simulink model "windEmulatorStep4_WECSim"  (R2025b)
settings: Solver=ode14x  StartTime=0  StopTime=400  FixedStep=Ts  MaxStep=0.01  RelTol=1e-3
values from neighbouring files (symbols this model uses):
  A = 1.0    (= 1)    [initStep4.m]
  absEncoderCountsToRad = 1/2^20*2*pi    (= 5.99211245268e-06)    [initStep4.m]
  acs800CtrlStruct =     [windEmulatorBusDefs.mat]
  acs800DcBusVoltsScaling = 1    [initStep4.m]
  acs800FreqScaling = 1/100    (= 0.01)    [initStep4.m]
  acs800PowerScaling = Gen_PowerScaling    (= 14.9109)    [initStep4.m]
  acs800SignalStruct =     [windEmulatorBusDefs.mat]
  acs800SpeedNomEng = 1500    [initStep4.m]
  acs800SpeedNomFb = 20000    [initStep4.m]
  acs800SpeedScaling = 1500/20000    (= 0.075)    [initStep4.m]
  acs800TempScaling = 1/10    (= 0.1)    [initStep4.m]
  acs800TorqueNomEng = 100    [initStep4.m]
  acs800TorqueNomFb = 10000    [initStep4.m]
  acs800TorqueScaling = acs800TorqueRating/10000    (= 0.008035933)    [initStep4.m]
  acs880CtrlStruct =     [windEmulatorBusDefs.mat]
  acs880FreqScaling = 60/20000    (= 0.003)    [initStep4.m]
  acs880MotorCurrentScaling = 100/10000    (= 0.01)    [initStep4.m]
  acs880MotorVoltsScaling = 1    [initStep4.m]
  acs880PowerScaling = 100*hp2W/10000    (= 7.457)    [initStep4.m]
  acs880RatedTorque = 80.494    [initStep4.m]
  acs880RateLimFalling = -10000    [initStep4.m]
  acs880RateLimRising = 10000    [initStep4.m]
  acs880SetpointLimLower = -0.975*acs880RatedTorque    (= -78.48165)    [initStep4.m]
  acs880SetpointLimUpper = 0.975*acs880RatedTorque    (= 78.48165)    [initStep4.m]
  acs880SignalStruct =     [windEmulatorBusDefs.mat]
  acs880SpeedPILimLo = -0.975*acs880RatedTorque    (= -78.48165)    [initStep4.m]
  acs880SpeedPILimUp = 0.975*acs880RatedTorque    (= 78.48165)    [initStep4.m]
  acs880SpeedScaling = 2000/20000    (= 0.1)    [initStep4.m]
  acs880TorqueFieldbusScale = 10000    [initStep4.m]
  acs880TorqueScaling = acs880RatedTorque/acs880TorqueFieldbusScale    (= 0.0080494)    [initStep4.m]
  acs880TorqueSetpointScaling = 100    [initStep4.m]
  bar2pa = 1e5    (= 100000)    [initStep4.m]
  belowMinPGain = 1/200    (= 0.005)    [initStep4.m]
  ctrlModeTorque = logical(true)    [init.m]    (also in initStep1.m; initStep2.m; initStep3.m; initStep4.m)
  ctrlSignal1 = squeeze(hptoSignalsData.Values.ctrlSignal1.Data)    [postProcessingStep2.m]
  ctrlSignal2 = squeeze(hptoSignalsData.Values.ctrlSignal2.Data)    [postProcessingStep2.m]
  deadBandController = boolean(false)    [initStep4.m]
  deadbandTorqueSlewRate = 300    [initStep4.m]
  Dm_max = 40    [initStep4.m]
  EffMechMax = 0.93    [initStep4.m]
  EffMechMin = 0.79    [initStep4.m]
  excForce_N = squeeze(hptoCtrlData.Values.excForce_N.Data)    [postProcessingStep2.m]
  expCtrlStruct =     [windEmulatorBusDefs.mat]
  FactorEff = psi2pa*cc2m3*(1/rev2rad)    (= 0.00109733470463)    [initStep4.m]
  fromFileSpeedSlewRate = 250    [initStep4.m]
  fromFileTorqueSlewRate = 25    [initStep4.m]
  futekTorqueScale = -1/(2^31)*10/5*100    (= -9.31322574615e-08)    [initStep4.m]
  genMaxTorque = 0.8*ratedTorque    (= 64.3952)    [initStep3.m]    (also in initStep4.m = 78.48165)
  genTorqueCmd_Nm = squeeze(hptoSignalsData.Values.genTorqueCmd_Nm.Data)    [postProcessingStep2.m]
  hbmCtScale = 1/1.5    (= 0.666666666667)    [initStep4.m]
  hbmPowerStruct =     [windEmulatorBusDefs.mat]
  hptoCtrlStruct =     [windEmulatorBusDefs.mat]
  hptoSignalStruct =     [windEmulatorBusDefs.mat]
  invPowerStruct =     [windEmulatorBusDefs.mat]
  lpm2m3ps = 1/m3ps2lpm    (= 1.66666666667e-05)    [initStep4.m]
  minPressureRef_psi = 1000    [initStep4.m]
  minTorqueRef_Nm = (minPressureRef_psi*psi2pa)*(Dm_max*cc2m3*(1/rev2rad))    (= 43.8933881851)    [initStep4.m]
  motorSpeed_rpm = squeeze(acs880SignalsData.Values.motorSpeed_rpm.Data)    [postProcessingStep2.m]
  nPreDrop = 2900    [initStep4.m]
  nPreDropMin = 725    [initStep4.m]
  psi2bar = 1/bar2psi    (= 0.0689475729318)    [initStep4.m]
  radps2rpm = 60/(2*pi)    (= 9.54929658551)    [initStep2.m]    (also in initStep4.m)
  rpm2radps = 2*pi/60    (= 0.10471975512)    [initStep4.m]
  runCounter = squeeze(hptoCtrlData.Values.runCounter.Data)    [postProcessingStep2.m]
  shaftSignalStruct =     [windEmulatorBusDefs.mat]
  sidCtrlStruct =     [windEmulatorBusDefs.mat]
  sidDataCaseCounter = sidData.experimentData.count    [initStep4.m]
  sidDataSpeed_rpm = sidData.experimentData.wShaft_rpm    [initStep4.m]
  sidDataTorque_Nm = sidData.experimentData.torqueShaft_Nm    [initStep4.m]
  sidInfoStruct =     [windEmulatorBusDefs.mat]
  T = 4    [initStep4.m]
  targetOmega = 2000/60*2*pi    (= 209.439510239)    [initStep2.m]    (also in initStep3.m; initStep4.m)
  time = hptoCtrlData.Values.runCounter.Time    [postProcessingStep2.m]
  TorqueLoadMax = 75    [initStep4.m]
  Ts = 1/250    (= 0.004)    [initStep4.m]
undefined symbols (not defined in the file or in its folder): absEncoderCounts, absEncoderPosition_rad, absEncoderSpeed_rpm, absEncoderStatus1, absEncoderStatus2, absEncoderTurns, accVolHP, acs800Torque_Nm, acs800TorqueSetpoint_Nm, acs880SpeedSetpoint_rpm, acs880Torque_Nm, body, constraint, crankLength, ctrlWord, dcBusVoltage_V, DiscIntNeverNeededParam, Dmax, excShaftSpeed_rpm, excShaftTorque_Nm, expType, expTypeEnum, frequency_Hz, fromFileCaseCounter, genPumpFlow_lpm, genShaftSpeed_rpm, genShaftSpeedRef, genSpeedActual, hmOutputShafTorque_Nm, iGainGen, m3persecond2lpm, motorCurrent_A, motorTorque_Nm, motorVoltage_V, offsetLength, pa2psi, pGainGen, pressure_bar, PressureControl, pto, radsec2rpm, ramp, resetHilIntegrator, resetSidIntegrator, rodLength, runHil, runSid, shaftPower_W, sidType, sidTypeEnum, SpeedControl, speedCtrlReset, speedRef_rpm, state, statusWord, stepCounter, temperature, torqueActual_Nm, TorqueInputControl, torqueSetpoint_Nm ... (+1)
libraries: slrealtimeethercatlib x118, fl_lib x81, nesl_utility x45, sh_lib x18, slrealtimeloglib x13, dspstat3 x5, slpidlib x4, simulink_extras x4, cstblocks x3, dspindex x3, WECSim_Lib_Body_Elements x2, simulink x2
(part 2 of 6)

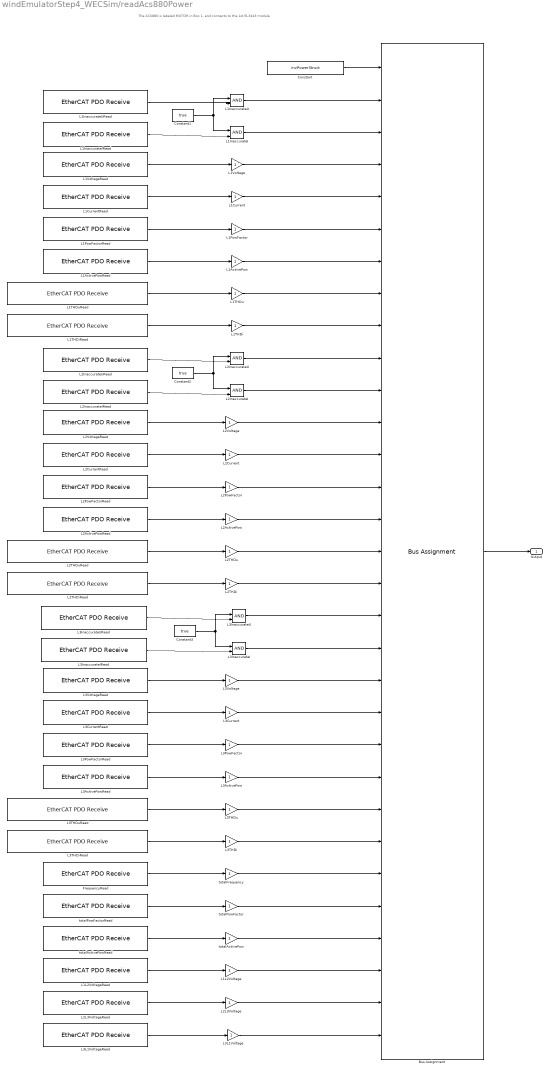
== system windEmulatorStep4_WECSim/readAcs880Power ==
  note: The ACS880 is labeled MOTOR in Box 1, and connects to the 1st EL3443 module
  Bus Assignment : BusAssignment  AssignedSignals=L1InaccurateU,L1InaccurateI,L1Voltage,L1Current,L1PowFactor,L1ActivePow,L1THDu,L1THDi,L2InaccurateU,L2InaccurateI,L2Voltage,L2Current,L2PowFactor,L2ActivePow,L2THDu,L2THDi,L3InaccurateU,L3InaccurateI,L3Voltage,L3Current,L3PowFactor,L3ActivePow,L3THDu,L3THDi,Frequency,TotalPowFactor,TotalActivePow,L1L2Voltage,L2L3Voltage,L3L1Volage
  Constant : Constant  Value=invPowerStruct  OutDataTypeStr=Bus: invPowerBus
  Constant1 : Constant  Value=true  OutDataTypeStr=boolean
  Constant2 : Constant  Value=true  OutDataTypeStr=boolean
  Constant3 : Constant  Value=true  OutDataTypeStr=boolean
  FrequencyRead : slrealtimeethercatlib/EtherCAT PDO Receive  Priority=2  sig_name=POW_EL3443_01.Total Basic.Frequency  sig_offset=2280  sig_type=single  type_size=32  sig_dim=1  device_id=0  sample_time=0.004000
  L1ActivePow : Gain  OutDataTypeStr=double
  L1ActivePowRead : slrealtimeethercatlib/EtherCAT PDO Receive  Priority=2  sig_name=POW_EL3443_01.L1 Power.Active Power  sig_offset=1064  sig_type=single  type_size=32  sig_dim=1  device_id=0  sample_time=0.004000
  L1Current : Gain  OutDataTypeStr=double
  L1CurrentRead : slrealtimeethercatlib/EtherCAT PDO Receive  Priority=2  sig_name=POW_EL3443_01.L1 Basic.Current  sig_offset=1032  sig_type=single  type_size=32  sig_dim=1  device_id=0  sample_time=0.004000
  L1InaccurateI : Logic  IconShape=distinctive  AllPortsSameDT=off  OutDataTypeStr=boolean
  L1InaccurateIRead : slrealtimeethercatlib/EtherCAT PDO Receive  Priority=2  sig_name=POW_EL3443_01.L1 Status.Inaccurate Current  sig_offset=988  sig_type=boolean  type_size=1  sig_dim=1  device_id=0  sample_time=0.004000
  L1InaccurateU : Logic  IconShape=distinctive  AllPortsSameDT=off  OutDataTypeStr=boolean
  L1InaccurateURead : slrealtimeethercatlib/EtherCAT PDO Receive  Priority=2  sig_name=POW_EL3443_01.L1 Status.Inaccurate Voltage  sig_offset=987  sig_type=boolean  type_size=1  sig_dim=1  device_id=0  sample_time=0.004000
  L1L2Voltage : Gain  OutDataTypeStr=double
  L1L2VoltageRead : slrealtimeethercatlib/EtherCAT PDO Receive  Priority=2  sig_name=POW_EL3443_01.Total L-L Voltage.L1-L2 Voltage  sig_offset=2600  sig_type=single  type_size=32  sig_dim=1  device_id=0  sample_time=0.004000
  L1PowFactor : Gain  OutDataTypeStr=double
  L1PowFactorRead : slrealtimeethercatlib/EtherCAT PDO Receive  Priority=2  sig_name=POW_EL3443_01.L1 Power.Power Factor  sig_offset=1160  sig_type=single  type_size=32  sig_dim=1  device_id=0  sample_time=0.004000
  L1THDi : Gain  OutDataTypeStr=double
  L1THDiRead : slrealtimeethercatlib/EtherCAT PDO Receive  Priority=2  sig_name=POW_EL3443_01.L1 Advanced.Current Total Harmonic Distortion  sig_offset=1336  sig_type=single  type_size=32  sig_dim=1  device_id=0  sample_time=0.004000
  L1THDu : Gain  OutDataTypeStr=double
  L1THDuRead : slrealtimeethercatlib/EtherCAT PDO Receive  Priority=2  sig_name=POW_EL3443_01.L1 Advanced.Voltage Total Harmonic Distortion  sig_offset=1272  sig_type=single  type_size=32  sig_dim=1  device_id=0  sample_time=0.004000
  L1Voltage : Gain  OutDataTypeStr=double
  L1VoltageRead : slrealtimeethercatlib/EtherCAT PDO Receive  Priority=2  sig_name=POW_EL3443_01.L1 Basic.Voltage  sig_offset=1000  sig_type=single  type_size=32  sig_dim=1  device_id=0  sample_time=0.004000
  L2ActivePow : Gain  OutDataTypeStr=double
  L2ActivePowRead : slrealtimeethercatlib/EtherCAT PDO Receive  Priority=2  sig_name=POW_EL3443_01.L2 Power.Active Power  sig_offset=1480  sig_type=single  type_size=32  sig_dim=1  device_id=0  sample_time=0.004000
  L2Current : Gain  OutDataTypeStr=double
  L2CurrentRead : slrealtimeethercatlib/EtherCAT PDO Receive  Priority=2  sig_name=POW_EL3443_01.L2 Basic.Current  sig_offset=1448  sig_type=single  type_size=32  sig_dim=1  device_id=0  sample_time=0.004000
  L2InaccurateI : Logic  IconShape=distinctive  AllPortsSameDT=off  OutDataTypeStr=boolean
  L2InaccurateIRead : slrealtimeethercatlib/EtherCAT PDO Receive  Priority=2  sig_name=POW_EL3443_01.L2 Status.Inaccurate Current  sig_offset=1404  sig_type=boolean  type_size=1  sig_dim=1  device_id=0  sample_time=0.004000
  L2InaccurateU : Logic  IconShape=distinctive  AllPortsSameDT=off  OutDataTypeStr=boolean
  L2InaccurateURead : slrealtimeethercatlib/EtherCAT PDO Receive  Priority=2  sig_name=POW_EL3443_01.L2 Status.Inaccurate Voltage  sig_offset=1403  sig_type=boolean  type_size=1  sig_dim=1  device_id=0  sample_time=0.004000
  L2L3Voltage : Gain  OutDataTypeStr=double
  L2L3VoltageRead : slrealtimeethercatlib/EtherCAT PDO Receive  Priority=2  sig_name=POW_EL3443_01.Total L-L Voltage.L2-L3 Voltage  sig_offset=2632  sig_type=single  type_size=32  sig_dim=1  device_id=0  sample_time=0.004000
  L2PowFactor : Gain  OutDataTypeStr=double
  L2PowFactorRead : slrealtimeethercatlib/EtherCAT PDO Receive  Priority=2  sig_name=POW_EL3443_01.L2 Power.Power Factor  sig_offset=1576  sig_type=single  type_size=32  sig_dim=1  device_id=0  sample_time=0.004000
  L2THDi : Gain  OutDataTypeStr=double
  L2THDiRead : slrealtimeethercatlib/EtherCAT PDO Receive  Priority=2  sig_name=POW_EL3443_01.L2 Advanced.Current Total Harmonic Distortion  sig_offset=1752  sig_type=single  type_size=32  sig_dim=1  device_id=0  sample_time=0.004000
  L2THDu : Gain  OutDataTypeStr=double
  L2THDuRead : slrealtimeethercatlib/EtherCAT PDO Receive  Priority=2  sig_name=POW_EL3443_01.L2 Advanced.Voltage Total Harmonic Distortion  sig_offset=1688  sig_type=single  type_size=32  sig_dim=1  device_id=0  sample_time=0.004000
  L2Voltage : Gain  OutDataTypeStr=double
  L2VoltageRead : slrealtimeethercatlib/EtherCAT PDO Receive  Priority=2  sig_name=POW_EL3443_01.L2 Basic.Voltage  sig_offset=1416  sig_type=single  type_size=32  sig_dim=1  device_id=0  sample_time=0.004000
  L3ActivePow : Gain  OutDataTypeStr=double
  L3ActivePowRead : slrealtimeethercatlib/EtherCAT PDO Receive  Priority=2  sig_name=POW_EL3443_01.L3 Power.Active Power  sig_offset=1896  sig_type=single  type_size=32  sig_dim=1  device_id=0  sample_time=0.004000
  L3Current : Gain  OutDataTypeStr=double
  L3CurrentRead : slrealtimeethercatlib/EtherCAT PDO Receive  Priority=2  sig_name=POW_EL3443_01.L3 Basic.Current  sig_offset=1864  sig_type=single  type_size=32  sig_dim=1  device_id=0  sample_time=0.004000
  L3InaccurateI : Logic  IconShape=distinctive  AllPortsSameDT=off  OutDataTypeStr=boolean
  L3InaccurateIRead : slrealtimeethercatlib/EtherCAT PDO Receive  Priority=2  sig_name=POW_EL3443_01.L3 Status.Inaccurate Current  sig_offset=1820  sig_type=boolean  type_size=1  sig_dim=1  device_id=0  sample_time=0.004000
  L3InaccurateU : Logic  IconShape=distinctive  AllPortsSameDT=off  OutDataTypeStr=boolean
  L3InaccurateURead : slrealtimeethercatlib/EtherCAT PDO Receive  Priority=2  sig_name=POW_EL3443_01.L3 Status.Inaccurate Voltage  sig_offset=1819  sig_type=boolean  type_size=1  sig_dim=1  device_id=0  sample_time=0.004000
  L3L1Voltage : Gain  OutDataTypeStr=double
  L3L1VoltageRead : slrealtimeethercatlib/EtherCAT PDO Receive  Priority=2  sig_name=POW_EL3443_01.Total L-L Voltage.L3-L1 Voltage  sig_offset=2664  sig_type=single  type_size=32  sig_dim=1  device_id=0  sample_time=0.004000
  L3PowFactor : Gain  OutDataTypeStr=double
  L3PowFactorRead : slrealtimeethercatlib/EtherCAT PDO Receive  Priority=2  sig_name=POW_EL3443_01.L3 Power.Power Factor  sig_offset=1992  sig_type=single  type_size=32  sig_dim=1  device_id=0  sample_time=0.004000
  L3THDi : Gain  OutDataTypeStr=double
  L3THDiRead : slrealtimeethercatlib/EtherCAT PDO Receive  Priority=2  sig_name=POW_EL3443_01.L3 Advanced.Current Total Harmonic Distortion  sig_offset=2168  sig_type=single  type_size=32  sig_dim=1  device_id=0  sample_time=0.004000
  L3THDu : Gain  OutDataTypeStr=double
  L3THDuRead : slrealtimeethercatlib/EtherCAT PDO Receive  Priority=2  sig_name=POW_EL3443_01.L3 Advanced.Voltage Total Harmonic Distortion  sig_offset=2104  sig_type=single  type_size=32  sig_dim=1  device_id=0  sample_time=0.004000
  L3Voltage : Gain  OutDataTypeStr=double
  L3VoltageRead : slrealtimeethercatlib/EtherCAT PDO Receive  Priority=2  sig_name=POW_EL3443_01.L3 Basic.Voltage  sig_offset=1832  sig_type=single  type_size=32  sig_dim=1  device_id=0  sample_time=0.004000
  totalActivePow : Gain  OutDataTypeStr=double
  totalActivePowRead : slrealtimeethercatlib/EtherCAT PDO Receive  Priority=2  sig_name=POW_EL3443_01.Total Active.Active Power  sig_offset=2376  sig_type=single  type_size=32  sig_dim=1  device_id=0  sample_time=0.004000
  totalFrequency : Gain  OutDataTypeStr=double
  totalPowFactor : Gain  OutDataTypeStr=double
  totalPowFactorRead : slrealtimeethercatlib/EtherCAT PDO Receive  Priority=2  sig_name=POW_EL3443_01.Total Basic.Power Factor  sig_offset=2312  sig_type=single  type_size=32  sig_dim=1  device_id=0  sample_time=0.004000
  Output : Outport  OutDataTypeStr=Bus: invPowerBus
  wires:
  L1VoltageRead/1 -> L1Voltage/1
  Constant/1 -> Bus Assignment/1
  Bus Assignment/1 -> Output/1
  L1Voltage/1 -> Bus Assignment/4
  L1CurrentRead/1 -> L1Current/1
  L1Current/1 -> Bus Assignment/5
  L1PowFactorRead/1 -> L1PowFactor/1
  L1PowFactor/1 -> Bus Assignment/6
  L1ActivePowRead/1 -> L1ActivePow/1
  L1ActivePow/1 -> Bus Assignment/7
  L1THDuRead/1 -> L1THDu/1
  L1THDu/1 -> Bus Assignment/8
  L1THDi/1 -> Bus Assignment/9
  L1THDiRead/1 -> L1THDi/1
  L2THDiRead/1 -> L2THDi/1
  L2THDi/1 -> Bus Assignment/17
  L2THDu/1 -> Bus Assignment/16
  L2THDuRead/1 -> L2THDu/1
  L2ActivePow/1 -> Bus Assignment/15
  L2ActivePowRead/1 -> L2ActivePow/1
  L2PowFactor/1 -> Bus Assignment/14
  L2PowFactorRead/1 -> L2PowFactor/1
  L2Current/1 -> Bus Assignment/13
  L2CurrentRead/1 -> L2Current/1
  L2Voltage/1 -> Bus Assignment/12
  L2VoltageRead/1 -> L2Voltage/1
  L3VoltageRead/1 -> L3Voltage/1
  L3Voltage/1 -> Bus Assignment/20
  L3CurrentRead/1 -> L3Current/1
  L3Current/1 -> Bus Assignment/21
  L3PowFactorRead/1 -> L3PowFactor/1
  L3PowFactor/1 -> Bus Assignment/22
  L3ActivePowRead/1 -> L3ActivePow/1
  L3ActivePow/1 -> Bus Assignment/23
  L3THDuRead/1 -> L3THDu/1
  L3THDu/1 -> Bus Assignment/24
  L3THDi/1 -> Bus Assignment/25
  L3THDiRead/1 -> L3THDi/1
  Constant1/1 -> L1InaccurateU/1, L1InaccurateI/1
  L1InaccurateU/1 -> Bus Assignment/2
  L1InaccurateURead/1 -> L1InaccurateU/2
  L1InaccurateI/1 -> Bus Assignment/3
  L1InaccurateIRead/1 -> L1InaccurateI/2
  Constant2/1 -> L2InaccurateU/1, L2InaccurateI/1
  L2InaccurateURead/1 -> L2InaccurateU/2
  L2InaccurateI/1 -> Bus Assignment/11
  L2InaccurateIRead/1 -> L2InaccurateI/2
  L2InaccurateU/1 -> Bus Assignment/10
  L3InaccurateU/1 -> Bus Assignment/18
  L3InaccurateI/1 -> Bus Assignment/19
  L3InaccurateIRead/1 -> L3InaccurateI/2
  Constant3/1 -> L3InaccurateU/1, L3InaccurateI/1
  L3InaccurateURead/1 -> L3InaccurateU/2
  FrequencyRead/1 -> totalFrequency/1
  totalFrequency/1 -> Bus Assignment/26
  totalPowFactorRead/1 -> totalPowFactor/1
  totalPowFactor/1 -> Bus Assignment/27
  totalActivePowRead/1 -> totalActivePow/1
  totalActivePow/1 -> Bus Assignment/28
  L1L2VoltageRead/1 -> L1L2Voltage/1
  L1L2Voltage/1 -> Bus Assignment/29
  L2L3Voltage/1 -> Bus Assignment/30
  L2L3VoltageRead/1 -> L2L3Voltage/1
  L3L1VoltageRead/1 -> L3L1Voltage/1
  L3L1Voltage/1 -> Bus Assignment/31

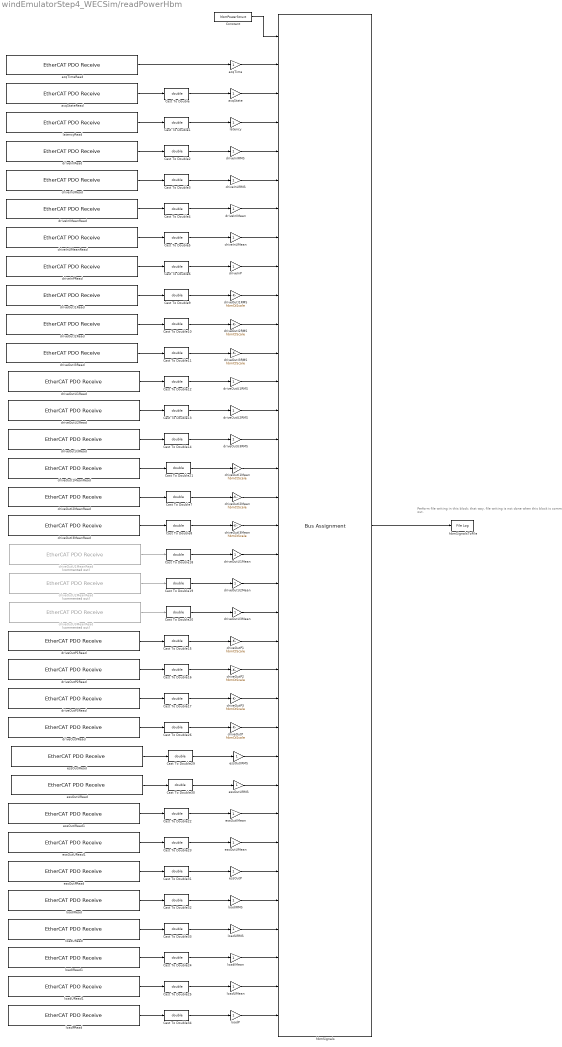
== system windEmulatorStep4_WECSim/readPowerHbm ==
  note: Perform file writing in this block; that way, file writing is not done when this block is commented out.
  Cast To Double{,1..26,29..34} (33 alike) : DataTypeConversion  OutDataTypeStr=double  SaturateOnIntegerOverflow=off  RndMeth=Floor
  Constant : Constant  Value=hbmPowerStruct  OutDataTypeStr=Bus: hbmPowerBus
  acqState : Gain  OutDataTypeStr=double
  acqStateRead : slrealtimeethercatlib/EtherCAT PDO Receive  Priority=2  sig_name=HBM_Power_Analyzer_01.AcquisitionState.AcquisitionState_S  sig_offset=4504  sig_type=uint8  type_size=8  sig_dim=1  device_id=0  sample_time=0.004000
  acqTime : Gain  OutDataTypeStr=double
  acqTimeRead : slrealtimeethercatlib/EtherCAT PDO Receive  Priority=2  sig_name=HBM_Power_Analyzer_01.AcquisitionTime.AcquisitionTime_V  sig_offset=4512  sig_type=double  type_size=64  sig_dim=1  device_id=0  sample_time=0.004000
  driveInIMean : Gain  OutDataTypeStr=double
  driveInIMeanRead : slrealtimeethercatlib/EtherCAT PDO Receive  Priority=2  sig_name=HBM_Power_Analyzer_01.Drive.in.i_mean.Drive.in.i_mean_V  sig_offset=4784  sig_type=single  type_size=32  sig_dim=1  device_id=0  sample_time=0.004000
  driveInIRMS : Gain  OutDataTypeStr=double
  driveInIRead : slrealtimeethercatlib/EtherCAT PDO Receive  Priority=2  sig_name=HBM_Power_Analyzer_01.Drive.in.I.Drive.in.I_V  sig_offset=4704  sig_type=single  type_size=32  sig_dim=1  device_id=0  sample_time=0.004000
  driveInP : Gain  OutDataTypeStr=double
  driveInPRead : slrealtimeethercatlib/EtherCAT PDO Receive  Priority=2  sig_name=HBM_Power_Analyzer_01.Drive.in.P.Drive.in.P_V  sig_offset=5104  sig_type=single  type_size=32  sig_dim=1  device_id=0  sample_time=0.004000
  driveInUMean : Gain  OutDataTypeStr=double
  driveInUMeanRead : slrealtimeethercatlib/EtherCAT PDO Receive  Priority=2  sig_name=HBM_Power_Analyzer_01.Drive.in.u_mean.Drive.in.u_mean_V  sig_offset=4824  sig_type=single  type_size=32  sig_dim=1  device_id=0  sample_time=0.004000
  driveInURMS : Gain  OutDataTypeStr=double
  driveInURead : slrealtimeethercatlib/EtherCAT PDO Receive  Priority=2  sig_name=HBM_Power_Analyzer_01.Drive.in.U.Drive.in.U_V  sig_offset=4744  sig_type=single  type_size=32  sig_dim=1  device_id=0  sample_time=0.004000
  driveOutI1Mean : Gain  Gain=hbmCtScale  OutDataTypeStr=double
  driveOutI1MeanRead : slrealtimeethercatlib/EtherCAT PDO Receive  Priority=2  sig_name=HBM_Power_Analyzer_01.Drive.out.i1_mean.Drive.out.i1_mean_V  sig_offset=5664  sig_type=single  type_size=32  sig_dim=1  device_id=0  sample_time=0.004000
  driveOutI1RMS : Gain  Gain=hbmCtScale  OutDataTypeStr=double
  driveOutI1Read : slrealtimeethercatlib/EtherCAT PDO Receive  Priority=2  sig_name=HBM_Power_Analyzer_01.Drive.out.I_1.Drive.out.I_1_V  sig_offset=4864  sig_type=single  type_size=32  sig_dim=1  device_id=0  sample_time=0.004000
  driveOutI2Mean : Gain  Gain=hbmCtScale  OutDataTypeStr=double
  driveOutI2MeanRead : slrealtimeethercatlib/EtherCAT PDO Receive  Priority=2  sig_name=HBM_Power_Analyzer_01.Drive.out.i2_mean.Drive.out.i2_mean_V  sig_offset=5704  sig_type=single  type_size=32  sig_dim=1  device_id=0  sample_time=0.004000
  driveOutI2RMS : Gain  Gain=hbmCtScale  OutDataTypeStr=double
  driveOutI2Read : slrealtimeethercatlib/EtherCAT PDO Receive  Priority=2  sig_name=HBM_Power_Analyzer_01.Drive.out.I_2.Drive.out.I_2_V  sig_offset=4904  sig_type=single  type_size=32  sig_dim=1  device_id=0  sample_time=0.004000
  driveOutI3Mean : Gain  Gain=hbmCtScale  OutDataTypeStr=double
  driveOutI3MeanRead : slrealtimeethercatlib/EtherCAT PDO Receive  Priority=2  sig_name=HBM_Power_Analyzer_01.Drive.out.i3_mean.Drive.out.i3_mean_V  sig_offset=5744  sig_type=single  type_size=32  sig_dim=1  device_id=0  sample_time=0.004000
  driveOutI3RMS : Gain  Gain=hbmCtScale  OutDataTypeStr=double
  driveOutI3Read : slrealtimeethercatlib/EtherCAT PDO Receive  Priority=2  sig_name=HBM_Power_Analyzer_01.Drive.out.I_3.Drive.out.I_3_V  sig_offset=5144  sig_type=single  type_size=32  sig_dim=1  device_id=0  sample_time=0.004000
  driveOutP{,1..3} (4 alike) : Gain  Gain=hbmCtScale  OutDataTypeStr=double
  driveOutP1Read : slrealtimeethercatlib/EtherCAT PDO Receive  Priority=2  sig_name=HBM_Power_Analyzer_01.Drive.out.P_1.Drive.out.P_1_V  sig_offset=5304  sig_type=single  type_size=32  sig_dim=1  device_id=0  sample_time=0.004000
  driveOutP2Read : slrealtimeethercatlib/EtherCAT PDO Receive  Priority=2  sig_name=HBM_Power_Analyzer_01.Drive.out.P_2.Drive.out.P_2_V  sig_offset=5344  sig_type=single  type_size=32  sig_dim=1  device_id=0  sample_time=0.004000
  driveOutP3Read : slrealtimeethercatlib/EtherCAT PDO Receive  Priority=2  sig_name=HBM_Power_Analyzer_01.Drive.out.P_3.Drive.out.P_3_V  sig_offset=5384  sig_type=single  type_size=32  sig_dim=1  device_id=0  sample_time=0.004000
  driveOutPRead : slrealtimeethercatlib/EtherCAT PDO Receive  Priority=2  sig_name=HBM_Power_Analyzer_01.Drive.out.P.Drive.out.P_V  sig_offset=5904  sig_type=single  type_size=32  sig_dim=1  device_id=0  sample_time=0.004000
  driveOutU1Mean : Gain  OutDataTypeStr=double
  driveOutU1MeanRead : slrealtimeethercatlib/EtherCAT PDO Receive  Priority=2  Commented=on  sig_name=HBM_Power_Analyzer_01.Drive_out.u1_mean.Drive_out.u1_mean_V  sig_offset=8208  sig_type=single  type_size=32  sig_dim=1  device_id=0  sample_time=0.001000
  driveOutU1RMS : Gain  OutDataTypeStr=double
  driveOutU1Read : slrealtimeethercatlib/EtherCAT PDO Receive  Priority=2  sig_name=HBM_Power_Analyzer_01.Drive.out.U_1.Drive.out.U_1_V  sig_offset=5184  sig_type=single  type_size=32  sig_dim=1  device_id=0  sample_time=0.004000
  driveOutU2Mean : Gain  OutDataTypeStr=double
  driveOutU2MeanRead : slrealtimeethercatlib/EtherCAT PDO Receive  Priority=2  Commented=on  sig_name=HBM_Power_Analyzer_01.Drive_out.u2_mean.Drive_out.u2_mean_V  sig_offset=8408  sig_type=single  type_size=32  sig_dim=1  device_id=0  sample_time=0.001000
  driveOutU2RMS : Gain  OutDataTypeStr=double
  driveOutU2Read : slrealtimeethercatlib/EtherCAT PDO Receive  Priority=2  sig_name=HBM_Power_Analyzer_01.Drive.out.U_2.Drive.out.U_2_V  sig_offset=5224  sig_type=single  type_size=32  sig_dim=1  device_id=0  sample_time=0.004000
  driveOutU3Mean : Gain  OutDataTypeStr=double
  driveOutU3MeanRead : slrealtimeethercatlib/EtherCAT PDO Receive  Priority=2  Commented=on  sig_name=HBM_Power_Analyzer_01.Drive_out.u3_mean.Drive_out.u3_mean_V  sig_offset=8448  sig_type=single  type_size=32  sig_dim=1  device_id=0  sample_time=0.001000
  driveOutU3RMS : Gain  OutDataTypeStr=double
  driveOutU3Read : slrealtimeethercatlib/EtherCAT PDO Receive  Priority=2  sig_name=HBM_Power_Analyzer_01.Drive.out.U_3.Drive.out.U_3_V  sig_offset=5264  sig_type=single  type_size=32  sig_dim=1  device_id=0  sample_time=0.004000
  essOutIMean : Gain  OutDataTypeStr=double
  essOutIRMS : Gain  OutDataTypeStr=double
  essOutIRead : slrealtimeethercatlib/EtherCAT PDO Receive  Priority=2  sig_name=HBM_Power_Analyzer_01.ESS.out1.I.ESS.out1.I_V  sig_offset=4624  sig_type=single  type_size=32  sig_dim=1  device_id=0  sample_time=0.004000
  essOutIRead1 : slrealtimeethercatlib/EtherCAT PDO Receive  Priority=2  sig_name=HBM_Power_Analyzer_01.ESS.out1.i_mean.ESS.out1.i_mean_V  sig_offset=5064  sig_type=single  type_size=32  sig_dim=1  device_id=0  sample_time=0.004000
  essOutP : Gain  OutDataTypeStr=double
  essOutPRead : slrealtimeethercatlib/EtherCAT PDO Receive  Priority=2  sig_name=HBM_Power_Analyzer_01.ESS.out1.P.ESS.out1.P_V  sig_offset=4944  sig_type=single  type_size=32  sig_dim=1  device_id=0  sample_time=0.004000
  essOutUMean : Gain  OutDataTypeStr=double
  essOutURMS : Gain  OutDataTypeStr=double
  essOutURead : slrealtimeethercatlib/EtherCAT PDO Receive  Priority=2  sig_name=HBM_Power_Analyzer_01.ESS.out1.U.ESS.out1.U_V  sig_offset=4664  sig_type=single  type_size=32  sig_dim=1  device_id=0  sample_time=0.004000
  essOutURead1 : slrealtimeethercatlib/EtherCAT PDO Receive  Priority=2  sig_name=HBM_Power_Analyzer_01.ESS.out1.u_mean.ESS.out1.u_mean_V  sig_offset=5544  sig_type=single  type_size=32  sig_dim=1  device_id=0  sample_time=0.004000
  hbmSignals : BusAssignment  AssignedSignals=acqTime,acqState,latency,driveInIRMS,driveInURMS,driveInIMean,driveInUMean,driveInP,driveOutI1RMS,driveOutI2RMS,driveOutI3RMS,driveOutU1RMS,driveOutU2RMS,driveOutU3RMS,driveOutI1Mean,driveOutI2Mean,driveOutI3Mean,driveOutU1Mean,driveOutU2Mean,driveOutU3Mean,driveOutP1,driveOutP2,driveOutP3,driveOutP,essOutIRMS,essOutURMS,essOutIMean,essOutUMean,essOutP,loadIRMS,loadURMS,loadIMean,loadUMean,loadP
  hbmSignalsToFile : slrealtimeloglib/File Log  decimation=fileDecimation  inputProcessing=Elements as channels (sample based)
  latency : Gain  OutDataTypeStr=double
  latencyRead : slrealtimeethercatlib/EtherCAT PDO Receive  Priority=2  sig_name=HBM_Power_Analyzer_01.Latency.Latency_V  sig_offset=4584  sig_type=single  type_size=32  sig_dim=1  device_id=0  sample_time=0.004000
  loadIMean : Gain  OutDataTypeStr=double
  loadIRMS : Gain  OutDataTypeStr=double
  loadIRead : slrealtimeethercatlib/EtherCAT PDO Receive  Priority=2  sig_name=HBM_Power_Analyzer_01.Load.in1.I.Load.in1.I_V  sig_offset=5424  sig_type=single  type_size=32  sig_dim=1  device_id=0  sample_time=0.004000
  loadIRead1 : slrealtimeethercatlib/EtherCAT PDO Receive  Priority=2  sig_name=HBM_Power_Analyzer_01.Load.in1.i_mean.Load.in1.i_mean_V  sig_offset=5584  sig_type=single  type_size=32  sig_dim=1  device_id=0  sample_time=0.004000
  loadP : Gain  OutDataTypeStr=double
  loadPRead : slrealtimeethercatlib/EtherCAT PDO Receive  Priority=2  sig_name=HBM_Power_Analyzer_01.Load.in1.P.Load.in1.P_V  sig_offset=5504  sig_type=single  type_size=32  sig_dim=1  device_id=0  sample_time=0.004000
  loadUMean : Gain  OutDataTypeStr=double
  loadURMS : Gain  OutDataTypeStr=double
  loadURead : slrealtimeethercatlib/EtherCAT PDO Receive  Priority=2  sig_name=HBM_Power_Analyzer_01.Load.in1.U.Load.in1.U_V  sig_offset=5464  sig_type=single  type_size=32  sig_dim=1  device_id=0  sample_time=0.004000
  loadURead1 : slrealtimeethercatlib/EtherCAT PDO Receive  Priority=2  sig_name=HBM_Power_Analyzer_01.Load.in1.u_mean.Load.in1.u_mean_V  sig_offset=5624  sig_type=single  type_size=32  sig_dim=1  device_id=0  sample_time=0.004000
  wires:
  acqTimeRead/1 -> acqTime/1
  acqTime/1 -> hbmSignals/2
  Constant/1 -> hbmSignals/1
  hbmSignals/1 -> hbmSignalsToFile/1
  Cast To Double/1 -> acqState/1
  acqState/1 -> hbmSignals/3
  latency/1 -> hbmSignals/4
  Cast To Double1/1 -> latency/1
  driveInIRead/1 -> Cast To Double2/1
  Cast To Double2/1 -> driveInIRMS/1
  driveInURead/1 -> Cast To Double3/1
  Cast To Double3/1 -> driveInURMS/1
  driveInIMeanRead/1 -> Cast To Double4/1
  Cast To Double4/1 -> driveInIMean/1
  driveInUMeanRead/1 -> Cast To Double5/1
  Cast To Double5/1 -> driveInUMean/1
  driveInPRead/1 -> Cast To Double6/1
  Cast To Double6/1 -> driveInP/1
  driveOutI1Read/1 -> Cast To Double9/1
  Cast To Double9/1 -> driveOutI1RMS/1
  driveOutI1RMS/1 -> hbmSignals/10
  driveOutI2Read/1 -> Cast To Double10/1
  Cast To Double10/1 -> driveOutI2RMS/1
  driveOutI2RMS/1 -> hbmSignals/11
  driveOutI3Read/1 -> Cast To Double11/1
  Cast To Double11/1 -> driveOutI3RMS/1
  driveOutI3RMS/1 -> hbmSignals/12
  driveOutU1Read/1 -> Cast To Double12/1
  Cast To Double12/1 -> driveOutU1RMS/1
  driveOutU1RMS/1 -> hbmSignals/13
  driveOutU2Read/1 -> Cast To Double13/1
  Cast To Double13/1 -> driveOutU2RMS/1
  driveOutU2RMS/1 -> hbmSignals/14
  driveOutU3Read/1 -> Cast To Double14/1
  Cast To Double14/1 -> driveOutU3RMS/1
  driveOutU3RMS/1 -> hbmSignals/15
  driveOutP1Read/1 -> Cast To Double15/1
  Cast To Double15/1 -> driveOutP1/1
  driveOutP1/1 -> hbmSignals/22
  driveOutP2Read/1 -> Cast To Double16/1
  Cast To Double16/1 -> driveOutP2/1
  driveOutP2/1 -> hbmSignals/23
  driveOutP3Read/1 -> Cast To Double17/1
  Cast To Double17/1 -> driveOutP3/1
  driveOutP3/1 -> hbmSignals/24
  driveOutPRead/1 -> Cast To Double26/1
  Cast To Double26/1 -> driveOutP/1
  driveOutP/1 -> hbmSignals/25
  essOutIRead/1 -> Cast To Double29/1
  Cast To Double29/1 -> essOutIRMS/1
  essOutURead/1 -> Cast To Double30/1
  Cast To Double30/1 -> essOutURMS/1
  essOutPRead/1 -> Cast To Double31/1
  Cast To Double31/1 -> essOutP/1
  essOutP/1 -> hbmSignals/30
  loadIRead/1 -> Cast To Double32/1
  Cast To Double32/1 -> loadIRMS/1
  loadURead/1 -> Cast To Double33/1
  Cast To Double33/1 -> loadURMS/1
  loadURMS/1 -> hbmSignals/32
  loadPRead/1 -> Cast To Double34/1
  Cast To Double34/1 -> loadP/1
  loadP/1 -> hbmSignals/35
  acqStateRead/1 -> Cast To Double/1
  latencyRead/1 -> Cast To Double1/1
  driveInIRMS/1 -> hbmSignals/5
  driveInURMS/1 -> hbmSignals/6
  driveInIMean/1 -> hbmSignals/7
  driveInUMean/1 -> hbmSignals/8
  driveInP/1 -> hbmSignals/9
  Cast To Double18/1 -> driveOutU1Mean/1
  driveOutI2MeanRead/1 -> Cast To Double7/1
  Cast To Double7/1 -> driveOutI2Mean/1
  driveOutU2MeanRead/1 -> Cast To Double19/1
  Cast To Double20/1 -> driveOutU3Mean/1
  driveOutI3MeanRead/1 -> Cast To Double8/1
  driveOutU1MeanRead/1 -> Cast To Double18/1
  driveOutU3MeanRead/1 -> Cast To Double20/1
  Cast To Double8/1 -> driveOutI3Mean/1
  driveOutI1MeanRead/1 -> Cast To Double21/1
  Cast To Double19/1 -> driveOutU2Mean/1
  Cast To Double21/1 -> driveOutI1Mean/1
  driveOutU3Mean/1 -> hbmSignals/21
  driveOutU2Mean/1 -> hbmSignals/20
  driveOutU1Mean/1 -> hbmSignals/19
  driveOutI3Mean/1 -> hbmSignals/18
  driveOutI2Mean/1 -> hbmSignals/17
  driveOutI1Mean/1 -> hbmSignals/16
  loadIRMS/1 -> hbmSignals/31
  essOutIRMS/1 -> hbmSignals/26
  essOutURMS/1 -> hbmSignals/27
  essOutIMean/1 -> hbmSignals/28
  essOutUMean/1 -> hbmSignals/29
  Cast To Double23/1 -> essOutUMean/1
  Cast To Double22/1 -> essOutIMean/1
  essOutURead1/1 -> Cast To Double23/1
  essOutIRead1/1 -> Cast To Double22/1
  loadUMean/1 -> hbmSignals/34
  loadURead1/1 -> Cast To Double25/1
  Cast To Double24/1 -> loadIMean/1
  loadIMean/1 -> hbmSignals/33
  loadIRead1/1 -> Cast To Double24/1
  Cast To Double25/1 -> loadUMean/1

== system windEmulatorStep4_WECSim/readShaftSignals ==
  note: Note: why is conversion to uint8 needed?
  Bus Assignment : BusAssignment  AssignedSignals=torqueActual_Nm,absEncoderCounts,absEncoderTurns,absEncoderPosition_rad,absEncoderSpeed_rpm,absEncoderStatus1,absEncoderStatus2
  Cast To Double : DataTypeConversion  OutDataTypeStr=double  SaturateOnIntegerOverflow=off  RndMeth=Floor
  Cast To Double1 : DataTypeConversion  OutDataTypeStr=uint8  SaturateOnIntegerOverflow=off  RndMeth=Floor
  Cast To Double2 : DataTypeConversion  OutDataTypeStr=uint8  SaturateOnIntegerOverflow=off  RndMeth=Floor
  Constant : Constant  Value=shaftSignalStruct  OutDataTypeStr=Bus: shaftSignalBus
  Demux : Demux  Outputs=2
  EtherCAT PDO Receive7 : slrealtimeethercatlib/EtherCAT PDO Receive  Priority=2  sig_name=InstA_EL5001_01.SSI Inputs.Status  sig_offset=936  sig_type=uint8  type_size=8  sig_dim=2  device_id=0  sample_time=0.004000
  Gain : Gain  Gain=futekTorqueScale
  countsToRads : Subsystem
  posToVel : simulink/Discrete/Discrete Derivative  gainval=1.0  ICPrevScaledInput=0.0  OutMin=[]  OutMax=[]  OutDataType=fixdt(1, 16)  OutScaling=2^-10  DoSatur=off
  rad/s->rpm : Gain  Gain=radps2rpm
  readEncoderCounter : slrealtimeethercatlib/EtherCAT PDO Receive  Priority=2  sig_name=InstA_EL5001_01.SSI Inputs.Counter value  sig_offset=952  sig_type=uint32  type_size=32  sig_dim=1  device_id=0  sample_time=0.004000
  readTorqueInput : slrealtimeethercatlib/EtherCAT PDO Receive  Priority=2  sig_name=InstA_EL3602_01.AI Inputs Channel 1.Value  sig_offset=856  sig_type=int32  type_size=32  sig_dim=1  device_id=0  sample_time=0.004000
  shaftSignals : Outport  OutDataTypeStr=Bus: shaftSignalBus
  wires:
  Bus Assignment/1 -> shaftSignals/1
  Constant/1 -> Bus Assignment/1
  readTorqueInput/1 -> Cast To Double/1
  Gain/1 -> Bus Assignment/2
  Demux/1 -> Cast To Double1/1
  Cast To Double/1 -> Gain/1
  Cast To Double1/1 -> Bus Assignment/7
  Demux/2 -> Cast To Double2/1
  Cast To Double2/1 -> Bus Assignment/8
  EtherCAT PDO Receive7/1 -> Demux/1  "encoderStatus"
  readEncoderCounter/1 -> countsToRads/1(rawCounts), Bus Assignment/3
  countsToRads/2(pos_rad) -> posToVel/1, Bus Assignment/5
  rad/s->rpm/1 -> Bus Assignment/6
  posToVel/1 -> rad/s->rpm/1
  countsToRads/1(turns) -> Bus Assignment/4

== system windEmulatorStep4_WECSim/sidCtrl ==
  expCtrl : Inport  OutDataTypeStr=Bus: expCtrlBus
  acs880Signals : Inport  Port=2  OutDataTypeStr=Bus: acs880SignalBus
  acs800Signals : Inport  Port=3  OutDataTypeStr=Bus: acs800SignalBus
  inportSpeed_rpm : Inport  Port=4
  inportTorque_Nm : Inport  Port=5
  inportCaseCounter : Inport  Port=6
  Bus Assignment : BusAssignment  AssignedSignals=acs800Torque_Nm,acs880Torque_Nm
  Bus Selector : BusSelector  OutputSignals=motorSpeed_rpm
  Bus Selector1 : BusSelector  OutputSignals=resetSidIntegrator
  Constant : Constant  Value=sidCtrlStruct  OutDataTypeStr=Bus: sidCtrlBus
  Constant1 : Constant  Value=acs880SpeedPILimUp
  Constant2 : Constant  Value=acs880SpeedPILimLo
  PID Controller : slpidlib/PID Controller  Controller=PI  Form=Parallel  TimeDomain=Continuous-time  UseExternalTs=off  SampleTime=-1  IntegratorMethod=Forward Euler  FilterMethod=Forward Euler  ControllerParametersSource=external  P=1  I=1  UseKiTs=off  D=0  UseExternalDerivativeSource=off  N=100  UseFilter=on  TunerSelectOption=Transfer Function Based (PID Tuner App)  InitialConditionSource=internal  InitialConditionForIntegrator=0  InitialConditionForFilter=0  DifferentiatorICPrevScaledInput=0  ExternalReset=level  TrackingMode=off  Kt=1  LimitOutput=on  SatLimitsSource=external  UpperSaturationLimit=inf  LowerSaturationLimit=-inf  LinearizeAsGain=on  AntiWindupMode=none  Kb=1  LimitIntegrator=off  UpperIntegratorSaturationLimit=inf  LowerIntegratorSaturationLimit=-inf  POutMin=[]  POutMax=[]  IOutMin=[]  IOutMax=[]  DOutMin=[]  DOutMax=[]  NOutMin=[]  NOutMax=[]  SumOutMin=[]  SumOutMax=[]  SaturationOutMin=[]  SaturationOutMax=[]  PParamMin=[]  PParamMax=[]  IParamMin=[]  IParamMax=[]  DParamMin=[]  DParamMax=[]  NParamMin=[]  NParamMax=[]  KbParamMin=[]  KbParamMax=[]  KtParamMin=[]  KtParamMax=[]  KbOutMin=[]  KbOutMax=[]  KtOutMin=[]  KtOutMax=[]  IntegratorOutMin=[]  IntegratorOutMax=[]  FilterOutMin=[]  FilterOutMax=[]  SumI1OutMin=[]  SumI1OutMax=[]  SumI2OutMin=[]  SumI2OutMax=[]  SumI3OutMin=[]  SumI3OutMax=[]  SumI4OutMin=[]  SumI4OutMax=[]  SumDOutMin=[]  SumDOutMax=[]  DifferentiatorOutMin=[]  DifferentiatorOutMax=[]  FilterDiffOutCoefMin=[]  FilterDiffOutCoefMax=[]  ReciprocalOutMin=[]  ReciprocalOutMax=[]  SumDenOutMin=[]  SumDenOutMax=[]  SumNumOutMin=[]  SumNumOutMax=[]  DivideOutMin=[]  DivideOutMax=[]  UdiffTsProdOutMin=[]  UdiffTsProdOutMax=[]  NTsProdOutMin=[]  NTsProdOutMax=[]  UintegralTsProdOutMin=[]  UintegralTsProdOutMax=[]  UngainTsProdOutMin=[]  UngainTsProdOutMax=[]  ClampingZeroOutDataTypeStr=Inherit: Inherit via back propagation  ClampingZeroOutMin=[]  ClampingZeroOutMax=[]  FilterDenConstantOutDataTypeStr=Inherit: Inherit via back propagation  FilterDenConstantOutMin=[]  FilterDenConstantOutMax=[]  PCopyOutDataTypeStr=Inherit: Inherit via back propagation  PCopyOutMin=[]  PCopyOutMax=[]  NCopyOutDataTypeStr=Inherit: Inherit via back propagation  NCopyOutMin=[]  NCopyOutMax=[]  IntegratorContinuousStateAttributes=''  IntegratorStateMustResolveToSignalObject=off  IntegratorRTWStateStorageClass=Auto  FilterContinuousStateAttributes=''  FilterStateMustResolveToSignalObject=off  FilterRTWStateStorageClass=Auto  ParallelPVariant=ExternalParameters  IdealPVariant=Disabled  IVariant=ExternalParameters  DVariant=Disabled  IntegratorVariant=Continuous  SatVariant=External  AWVariant=Passthrough  PCopyVariant=Disabled  TRVariant=Disabled  FdbkBlocksVariant=Forward  IdealPFdbkVariant=Disabled  SatFdbkVariant=Disabled  DerivativeFilterVariant=Disabled  NVariant=Disabled  NCopyVariant=Disabled_SignalSpec  FilterICVariant=Disabled  IntegratorICVariant=InternalICs  ExternalResetVariant=ExternalReset  TRSumVariant=Passthrough  SumFdbkVariant=Disabled  SumVariant=Sum_PI  TsampFilterVariant=InternalTs  TsampNgainVariant=Passthrough  TsampIntegralVariant=Disabled_SignalSpec  ExternalSaturationOutDataTypeStr=Inherit: Same as second input  DerivativeSourceVariant=Disabled  PreIntVariant=InternalPreInt
  Sum : Sum  Inputs=|+-
  Terminator1 : Terminator
  acs880SpeedIGain : Constant  Value=0
  acs880SpeedPGain : Constant  Value=0
  setpointGenerator : Subsystem
  sidCtrlSignals : Outport  OutDataTypeStr=Bus: sidCtrlBus
  sidInfoSignals : Outport  Port=2  OutDataTypeStr=Bus: sidInfoBus
  wires:
  Constant/1 -> Bus Assignment/1
  Bus Assignment/1 -> sidCtrlSignals/1
  acs800Signals/1 -> Terminator1/1
  acs880Signals/1 -> Bus Selector/1
  setpointGenerator/2(acs880SpeedSetpoint_rpm) -> Sum/1
  Bus Selector/1 -> Sum/2  "<motorSpeed_rpm>"
  setpointGenerator/1(acs800TorqueSetpoint_Nm) -> Bus Assignment/2
  Sum/1 -> PID Controller/1
  PID Controller/1 -> Bus Assignment/3
  acs880SpeedPGain/1 -> PID Controller/2
  acs880SpeedIGain/1 -> PID Controller/3
  expCtrl/1 -> Bus Selector1/1, setpointGenerator/1(expCtrl)
  Bus Selector1/1 -> PID Controller/4  "<resetSidIntegrator>"
  Constant1/1 -> PID Controller/5
  Constant2/1 -> PID Controller/6
  setpointGenerator/3(sidInfoSignals) -> sidInfoSignals/1
  inportSpeed_rpm/1 -> setpointGenerator/2(inportSpeed_rpm)
  inportTorque_Nm/1 -> setpointGenerator/3(inportTorque_Nm)
  inportCaseCounter/1 -> setpointGenerator/4(inportCaseCounter)

== system windEmulatorStep4_WECSim/writeAcs800Pdos ==
  note: Set to zero; we are in torque control.
  acs800CtrlSignals : Inport  OutDataTypeStr=Bus: acs800CtrlBus
  ACS800ConvertREF1 : Subsystem  mask{EngineeringValue=acs800SpeedNomEng, FieldbusValue=acs800SpeedNomFb}
      mask prompts: EngineeringValue "Engineering units nominal value:"; FieldbusValue "Fieldbus nominal value:"
  ACS800ConvertREF2 : Subsystem  mask{EngineeringValue=acs800TorqueNomEng, FieldbusValue=acs800TorqueNomFb}
      mask prompts: EngineeringValue "Engineering units nominal value:"; FieldbusValue "Fieldbus nominal value:"
  ACS800CtrlWord : slrealtimeethercatlib/EtherCAT PDO Transmit  Priority=3  sig_name=ACS800.RxPDO 1.ControlWord (Transparent)  sig_offset=520  sig_type=uint16  type_size=16  sig_dim=1  device_id=0  sample_time=0.004000
  ACS800Ref1Int16 : DataTypeConversion  OutDataTypeStr=int16  SaturateOnIntegerOverflow=off  RndMeth=Floor
  ACS800Ref2Int16 : DataTypeConversion  OutDataTypeStr=int16  SaturateOnIntegerOverflow=off  RndMeth=Floor
  ACS800SpeedSetpoint : slrealtimeethercatlib/EtherCAT PDO Transmit  Priority=3  sig_name=ACS800.RxPDO 1.REF1 (Speed)  sig_offset=536  sig_type=int16  type_size=16  sig_dim=1  device_id=0  sample_time=0.004000
  ACS800TorqueSetpoint : slrealtimeethercatlib/EtherCAT PDO Transmit  Priority=3  sig_name=ACS800.RxPDO 1.REF2 (Torque)  sig_offset=552  sig_type=int16  type_size=16  sig_dim=1  device_id=0  sample_time=0.004000
  Bus Selector : BusSelector  OutputSignals=ctrlWord,torqueSetpoint_percent
  Constant : Constant  Value=0
  wires:
  Constant/1 -> ACS800ConvertREF1/1(Eng)
  ACS800ConvertREF1/1(Fb) -> ACS800Ref1Int16/1
  ACS800Ref2Int16/1 -> ACS800TorqueSetpoint/1
  ACS800ConvertREF2/1(Fb) -> ACS800Ref2Int16/1
  ACS800Ref1Int16/1 -> ACS800SpeedSetpoint/1
  acs800CtrlSignals/1 -> Bus Selector/1
  Bus Selector/1 -> ACS800CtrlWord/1  "<ctrlWord>"
  Bus Selector/2 -> ACS800ConvertREF2/1(Eng)  "<torqueSetpoint_percent>"

== system windEmulatorStep4_WECSim/writeAcs880Pdos ==
  note: Zero Speed setpoint (we are using torque control)
  acs880CtrlSignals : Inport  OutDataTypeStr=Bus: acs880CtrlBus
  ACS880ConvertREF2 : Subsystem  mask{EngineeringValue=acs880TorqueSetpointScaling, FieldbusValue=acs880TorqueFieldbusScale}
      mask prompts: EngineeringValue "Engineering units nominal value:"; FieldbusValue "Fieldbus nominal value:"
  ACS880CtrlWord : slrealtimeethercatlib/EtherCAT PDO Transmit  Priority=3  sig_name=ACS880.RxPDO 1.ABB Drives Control Word  sig_offset=344  sig_type=uint16  type_size=16  sig_dim=1  device_id=0  sample_time=0.004000
  ACS880Ref1Int16 : DataTypeConversion  OutDataTypeStr=int16  SaturateOnIntegerOverflow=off  RndMeth=Floor
  ACS880Ref2Int16 : DataTypeConversion  OutDataTypeStr=int16  SaturateOnIntegerOverflow=off  RndMeth=Floor
  ACS880SpeedSetpoint : slrealtimeethercatlib/EtherCAT PDO Transmit  Priority=3  sig_name=ACS880.RxPDO 1.ABB Drives REF1  sig_offset=360  sig_type=int16  type_size=16  sig_dim=1  device_id=0  sample_time=0.004000
  ACS880TorqueSetpoint : slrealtimeethercatlib/EtherCAT PDO Transmit  Priority=3  sig_name=ACS880.RxPDO 1.ABB Drives REF2  sig_offset=376  sig_type=int16  type_size=16  sig_dim=1  device_id=0  sample_time=0.004000
  Bus Selector : BusSelector  OutputSignals=ctrlWord,torqueSetpoint_percent
  Constant2 : Constant  Value=0
  wires:
  ACS880Ref2Int16/1 -> ACS880TorqueSetpoint/1
  ACS880ConvertREF2/1(Fb) -> ACS880Ref2Int16/1
  Constant2/1 -> ACS880Ref1Int16/1
  ACS880Ref1Int16/1 -> ACS880SpeedSetpoint/1
  Bus Selector/2 -> ACS880ConvertREF2/1(Eng)  "<torqueSetpoint_percent>"
  acs880CtrlSignals/1 -> Bus Selector/1
  Bus Selector/1 -> ACS880CtrlWord/1  "<ctrlWord>"

== system windEmulatorStep4_WECSim/acs800Ctrl/ACS880FieldbusControl ==
  powerUp : Inport  OutDataTypeStr=boolean
  powerDown : Inport  Port=2  OutDataTypeStr=boolean
  resetFault : Inport  Port=3  OutDataTypeStr=double
  eStop : Inport  Port=4  OutDataTypeStr=boolean
  StatusWord : Inport  Port=5
  ctrlMode : Inport  Port=6
  ABB Fieldbus Control : Stateflow chart  TreatAsAtomicUnit=on
  ControlWord : Outport
  state : Outport  Port=2
  wires:
  StatusWord/1 -> ABB Fieldbus Control/5(StatusWord)
  ABB Fieldbus Control/2(state) -> state/1
  resetFault/1 -> ABB Fieldbus Control/3(resetFault)
  powerUp/1 -> ABB Fieldbus Control/1(powerUp)
  powerDown/1 -> ABB Fieldbus Control/2(powerDown)
  ABB Fieldbus Control/1(ControlWord) -> ControlWord/1
  eStop/1 -> ABB Fieldbus Control/4(eStop)
  ctrlMode/1 -> ABB Fieldbus Control/6(cwEXT_CTRL_LOC)

== system windEmulatorStep4_WECSim/acs880Ctrl/ACS880FieldbusControl ==
  powerUp : Inport  OutDataTypeStr=boolean
  powerDown : Inport  Port=2  OutDataTypeStr=boolean
  resetFault : Inport  Port=3  OutDataTypeStr=double
  eStop : Inport  Port=4  OutDataTypeStr=boolean
  StatusWord : Inport  Port=5
  ctrlMode : Inport  Port=6
  ABB Fieldbus Control : Stateflow chart  TreatAsAtomicUnit=on
  ControlWord : Outport
  state : Outport  Port=2
  wires:
  StatusWord/1 -> ABB Fieldbus Control/5(StatusWord)
  ABB Fieldbus Control/2(state) -> state/1
  resetFault/1 -> ABB Fieldbus Control/3(resetFault)
  powerUp/1 -> ABB Fieldbus Control/1(powerUp)
  powerDown/1 -> ABB Fieldbus Control/2(powerDown)
  ABB Fieldbus Control/1(ControlWord) -> ControlWord/1
  eStop/1 -> ABB Fieldbus Control/4(eStop)
  ctrlMode/1 -> ABB Fieldbus Control/6(cwEXT_CTRL_LOC)

== system windEmulatorStep4_WECSim/fileAndUI/acs800CtrlSignalsUI ==
  acs800CtrlSignals : Inport  OutDataTypeStr=Bus: acs800CtrlBus
  Bus Selector : BusSelector  OutputSignals=ctrlWord,state,torqueSetpoint_Nm,torqueSetpoint_percent
  Terminator{,1..3} (4 alike) : Terminator
  ctrlWord : Bias  SaturateOnIntegerOverflow=off
  ctrlWordDetail : Subsystem
  state : Bias  SaturateOnIntegerOverflow=off
  torqueSetpoint_Nm : Gain
  torqueSetpoint_percent : Gain
  wires:
  acs800CtrlSignals/1 -> Bus Selector/1
  Bus Selector/1 -> ctrlWordDetail/1(<ctrlWord>), ctrlWord/1  "<ctrlWord>"
  ctrlWord/1 -> Terminator/1
  Bus Selector/2 -> state/1  "<state>"
  state/1 -> Terminator1/1
  Bus Selector/4 -> torqueSetpoint_percent/1  "<torqueSetpoint_percent>"
  torqueSetpoint_percent/1 -> Terminator2/1
  Bus Selector/3 -> torqueSetpoint_Nm/1  "<torqueSetpoint_Nm>"
  torqueSetpoint_Nm/1 -> Terminator3/1

== system windEmulatorStep4_WECSim/fileAndUI/acs800SignalsUI ==
  acs800Signals : Inport  OutDataTypeStr=Bus: acs800SignalBus
  Bus Selector : BusSelector  OutputSignals=dcBusVoltage_V,frequency_Hz,temperature,motorSpeed_rpm,motorTorque_Nm,shaftPower_W,statusWord
  Terminator{,1..6} (7 alike) : Terminator
  dcBusVoltage_V : Gain
  frequency_Hz : Gain
  motorSpeed_rpm : Gain
  motorTorque_Nm : Gain
  powerCals : Subsystem
  shaftPower_W : Gain
  statusWord : Bias  SaturateOnIntegerOverflow=off
  statusWordDetail : Subsystem
  temperature : Gain
  wires:
  acs800Signals/1 -> powerCals/1(acs800Signals), Bus Selector/1
  Bus Selector/1 -> dcBusVoltage_V/1  "<dcBusVoltage_V>"
  dcBusVoltage_V/1 -> Terminator/1
  Bus Selector/2 -> frequency_Hz/1  "<frequency_Hz>"
  frequency_Hz/1 -> Terminator1/1
  Bus Selector/3 -> temperature/1  "<temperature>"
  temperature/1 -> Terminator2/1
  Bus Selector/4 -> motorSpeed_rpm/1  "<motorSpeed_rpm>"
  motorSpeed_rpm/1 -> Terminator3/1
  Bus Selector/5 -> motorTorque_Nm/1  "<motorTorque_Nm>"
  motorTorque_Nm/1 -> Terminator4/1
  Bus Selector/6 -> shaftPower_W/1  "<shaftPower_W>"
  shaftPower_W/1 -> Terminator5/1
  Bus Selector/7 -> statusWordDetail/1(statusWord), statusWord/1  "<statusWord>"
  statusWord/1 -> Terminator6/1

== system windEmulatorStep4_WECSim/fileAndUI/acs880CtrlSignalsUI ==
  acs880CtrlSignals1 : Inport  OutDataTypeStr=Bus: acs880CtrlBus
  Bus Selector : BusSelector  OutputSignals=ctrlWord,state,torqueSetpoint_Nm,torqueSetpoint_percent
  Terminator{,1..3} (4 alike) : Terminator
  ctrlWord : Bias  SaturateOnIntegerOverflow=off
  ctrlWordDetail : Subsystem
  state : Bias  SaturateOnIntegerOverflow=off
  torqueSetpoint_Nm : Gain
  torqueSetpoint_percent : Gain
  wires:
  acs880CtrlSignals1/1 -> Bus Selector/1
  Bus Selector/1 -> ctrlWordDetail/1(<ctrlWord>), ctrlWord/1  "<ctrlWord>"
  ctrlWord/1 -> Terminator/1
  Bus Selector/2 -> state/1  "<state>"
  state/1 -> Terminator1/1
  Bus Selector/4 -> torqueSetpoint_percent/1  "<torqueSetpoint_percent>"
  torqueSetpoint_percent/1 -> Terminator2/1
  Bus Selector/3 -> torqueSetpoint_Nm/1  "<torqueSetpoint_Nm>"
  torqueSetpoint_Nm/1 -> Terminator3/1

== system windEmulatorStep4_WECSim/fileAndUI/acs880SignalsUI ==
  acs880Signals : Inport  OutDataTypeStr=Bus: acs880SignalBus
  Bus Selector : BusSelector  OutputSignals=motorVoltage_V,motorCurrent_A,frequency_Hz,motorSpeed_rpm,motorTorque_Nm,shaftPower_W,statusWord
  Terminator{,1..6} (7 alike) : Terminator
  frequency_Hz : Gain
  motorCurrent_A : Gain
  motorSpeed_rpm : Gain
  motorTorque_Nm : Gain
  motorVoltage_V : Gain
  powerCals : Subsystem
  shaftPower_W : Gain
  statusWord : Bias  SaturateOnIntegerOverflow=off
  statusWordDetail : Subsystem
  wires:
  acs880Signals/1 -> powerCals/1(acs880Signals), Bus Selector/1
  Bus Selector/1 -> motorVoltage_V/1  "<motorVoltage_V>"
  motorVoltage_V/1 -> Terminator/1
  Bus Selector/2 -> motorCurrent_A/1  "<motorCurrent_A>"
  motorCurrent_A/1 -> Terminator1/1
  Bus Selector/3 -> frequency_Hz/1  "<frequency_Hz>"
  frequency_Hz/1 -> Terminator2/1
  Bus Selector/4 -> motorSpeed_rpm/1  "<motorSpeed_rpm>"
  motorSpeed_rpm/1 -> Terminator3/1
  Bus Selector/5 -> motorTorque_Nm/1  "<motorTorque_Nm>"
  motorTorque_Nm/1 -> Terminator4/1
  Bus Selector/6 -> shaftPower_W/1  "<shaftPower_W>"
  shaftPower_W/1 -> Terminator5/1
  Bus Selector/7 -> statusWordDetail/1(statusWord), statusWord/1  "<statusWord>"
  statusWord/1 -> Terminator6/1

== system windEmulatorStep4_WECSim/fileAndUI/diagnostics ==
  Data Type Conversion : DataTypeConversion  OutDataTypeStr=double  SaturateOnIntegerOverflow=off  RndMeth=Floor
  Memory : Memory
  Sum : Sum  Inputs=|++  OutDataTypeStr=uint32
  Terminator : Terminator
  loopAdd : Constant  OutDataTypeStr=uint32
  loopCounter : Gain  ParamDataTypeStr=uint32  OutDataTypeStr=uint32
  time_s : Gain  Gain=Ts
  wires:
  loopCounter/1 -> Data Type Conversion/1
  Sum/1 -> loopCounter/1, Memory/1
  time_s/1 -> Terminator/1  "time_s"
  Memory/1 -> Sum/2
  Data Type Conversion/1 -> time_s/1
  loopAdd/1 -> Sum/1
